simulink model "LF_V15_Delay_Perfect"  (Simulink 7.9)
settings: Solver=ode45  StartTime=0.0  StopTime=100*20e-9  RelTol=1e-3
PreLoadFcn:
  | LF_V15_Param;
values from neighbouring files (symbols this model uses):
  Cnt_CPS = 10    [LF_V15_Param.m]
  Exp_ST = 1/Exp_SF    (= 0.002)    [LF_V15_Param.m]
  Kd2 = 0.004    [LF_V15_Param.m]
  Ki2 = 0.03    [LF_V15_Param.m]
  Kp2 = 0.25    [LF_V15_Param.m]
  Reg_En = (2^Err_Acc_Len)-1    (= 511)    [LF_V15_Param.m]
  Saw_CPS = 100    [LF_V15_Param.m]
libraries: xbsIndex_r4 x273
(part 2 of 2)

== system LF_V15_Delay_Perfect/DC_Direction_Controller/Sampler/Pulse_generator ==
  Freq : Inport
  Accumulator1 : xbsIndex_r4/Accumulator  operation=Add  n_bits=26  overflow=Wrap  scale=1  rst=on  infoeditControl=reset for floating point data type must be asserted for a minimum of 2 cycles  hasbypass=off  en=off  latency=0  dbl_ovrd=off  msb_inp=100  msb=100  lsb=-100  use_behavioral_HDL=on  implementation=Fabric  block_type=accum
  Constant5 : xbsIndex_r4/Constant  const=1/Exp_ST  gui_display_data_type=Fixed-point  arith_type=Unsigned  n_bits=26  bin_pt=0  preci_type=Single  exp_width=8  frac_width=24  explicit_period=on  period=Exp_ST  equ=P=C  opselect=C  inp2=PCIN>>17  opr=+  inp1=P  carry=CIN  dbl_ovrd=off  block_type=constant
  Relational1 : xbsIndex_r4/Relational  mode=a<=b  en=off  latency=0  dbl_ovrd=off  block_type=relational
  Pulse_Level : Outport
  wires:
  Freq/1 -> Accumulator1/1
  Constant5/1 -> Relational1/1
  Accumulator1/1 -> Relational1/2
  Relational1/1 -> Accumulator1/2, Pulse_Level/1

== system LF_V15_Delay_Perfect/DC_Direction_Controller/Sampler/Subsystem1 ==
  In1 : Inport
  Delay : xbsIndex_r4/Delay  rst=off  infoeditControl=Selection of Reset will increase slice count due to use of real FFs and instead of SRLs  en=off  latency=1  dbl_ovrd=off  reg_retiming=on  block_type=delay
  Inverter : xbsIndex_r4/Inverter  en=off  latency=0  dbl_ovrd=off  block_type=inv
  Logical : xbsIndex_r4/Logical  logical_function=AND  inputs=2  en=off  latency=0  precision=User Defined  arith_type=Unsigned  n_bits=1  bin_pt=0  align_bp=on  dbl_ovrd=off  block_type=logical
  Out1 : Outport
  wires:
  Delay/1 -> Logical/2
  Inverter/1 -> Delay/1
  In1/1 -> Logical/1, Inverter/1
  Logical/1 -> Out1/1

== system LF_V15_Delay_Perfect/RM_LM : Actuators/RM_LM: F_R_PWM_Generator/Sawtooth_generator ==
  Freq : Inport
  Accumulator1 : xbsIndex_r4/Accumulator  operation=Add  n_bits=28  overflow=Wrap  scale=1  rst=on  infoeditControl=reset for floating point data type must be asserted for a minimum of 2 cycles  hasbypass=off  en=off  latency=0  dbl_ovrd=off  msb_inp=100  msb=100  lsb=-100  use_behavioral_HDL=on  implementation=Fabric  block_type=accum
  Constant5 : xbsIndex_r4/Constant  const=1/Exp_ST  gui_display_data_type=Fixed-point  arith_type=Unsigned  n_bits=27  bin_pt=0  preci_type=Single  exp_width=8  frac_width=24  explicit_period=on  period=Exp_ST  equ=P=C  opselect=C  inp2=PCIN>>17  opr=+  inp1=P  carry=CIN  dbl_ovrd=off  block_type=constant
  Relational1 : xbsIndex_r4/Relational  mode=a<=b  en=off  latency=0  dbl_ovrd=off  block_type=relational
  Scaling_to_1 : xbsIndex_r4/CMult  const=Exp_ST  gui_display_data_type=Fixed-point  const_n_bits=43  const_bin_pt=43  float_type=Single  exp_bits=8  fraction_bits=24  en=off  latency=0  precision=User Defined  arith_type=Unsigned  n_bits=21  bin_pt=20  quantization=Truncate  overflow=Wrap  dbl_ovrd=off  use_behavioral_HDL=on  mem_type=Distributed RAM  pipeline=off  block_type=cmult
  Sawtooth : Outport
  wires:
  Relational1/1 -> Accumulator1/2
  Accumulator1/1 -> Relational1/2, Scaling_to_1/1
  Constant5/1 -> Relational1/1
  Freq/1 -> Accumulator1/1
  Scaling_to_1/1 -> Sawtooth/1

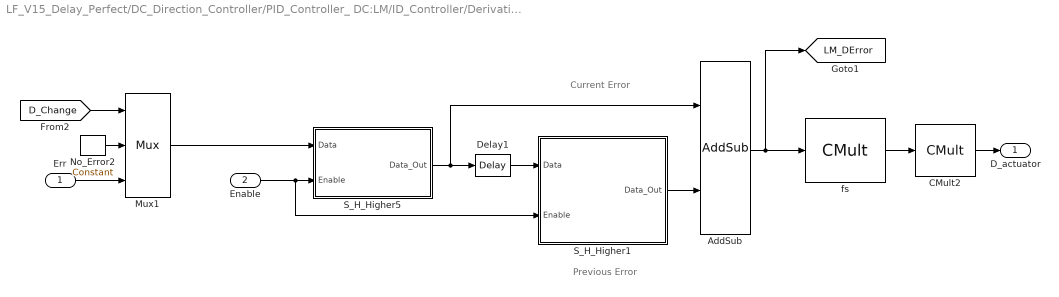
== system LF_V15_Delay_Perfect/DC_Direction_Controller/PID_Controller_ DC:LM/ID_Controller/Derivative ==
  note: Current Error
  note: Previous Error
  Err : Inport
  Enable : Inport  Port=2
  AddSub : xbsIndex_r4/AddSub  mode=Subtraction  use_carryin=off  use_carryout=off  en=off  latency=0  precision=User Defined  arith_type="Signed  (2's comp)"  n_bits=5  bin_pt=0  quantization=Truncate  overflow=Wrap  dbl_ovrd=off  use_behavioral_HDL=off  hw_selection=Fabric  pipelined=off  block_type=addsub
  CMult2 : xbsIndex_r4/CMult  const=Kd2  gui_display_data_type=Fixed-point  const_n_bits=8  const_bin_pt=8  float_type=Single  exp_bits=8  fraction_bits=24  en=off  latency=0  precision=User Defined  arith_type="Signed  (2's comp)"  n_bits=12  bin_pt=12  quantization=Truncate  overflow=Wrap  dbl_ovrd=off  use_behavioral_HDL=off  mem_type=Distributed RAM  pipeline=off  block_type=cmult
  Delay1 : xbsIndex_r4/Delay  rst=off  infoeditControl=Selection of Reset will increase slice count due to use of real FFs and instead of SRLs  en=off  latency=1  dbl_ovrd=off  reg_retiming=off  block_type=delay
  Mux1 : xbsIndex_r4/Mux  inputs=2  en=off  latency=0  precision=Full  arith_type="Signed  (2's comp)"  n_bits=25  bin_pt=20  quantization=Truncate  overflow=Wrap  dbl_ovrd=off  block_type=mux
  No_Error2 : xbsIndex_r4/Constant  const=0  gui_display_data_type=Fixed-point  arith_type=Unsigned  n_bits=1  bin_pt=0  preci_type=Single  exp_width=8  frac_width=24  explicit_period=on  period=Exp_ST  equ=P=C  opselect=C  inp2=PCIN>>17  opr=+  inp1=P  carry=CIN  dbl_ovrd=off  block_type=constant
  S_H_Higher1 : Subsystem
  S_H_Higher5 : Subsystem
  fs : xbsIndex_r4/CMult  const=Cnt_CPS  gui_display_data_type=Fixed-point  const_n_bits=4  const_bin_pt=0  float_type=Single  exp_bits=8  fraction_bits=24  en=off  latency=0  precision=User Defined  arith_type="Signed  (2's comp)"  n_bits=8  bin_pt=0  quantization=Truncate  overflow=Wrap  dbl_ovrd=off  use_behavioral_HDL=on  mem_type=Distributed RAM  pipeline=off  block_type=cmult
  D_actuator : Outport
  tag scope: LM_DError=global
  wires:
  CMult2/1 -> D_actuator/1
  fs/1 -> CMult2/1
  S_H_Higher5/1(Data_Out) -> AddSub/1, Delay1/1
  Enable/1 -> S_H_Higher1/2(Enable), S_H_Higher5/2(Enable)
  Delay1/1 -> S_H_Higher1/1(Data)
  S_H_Higher1/1(Data_Out) -> AddSub/2
  AddSub/1 -> fs/1, [LM_DError]
  [D_Change] -> Mux1/1
  Err/1 -> Mux1/3
  Mux1/1 -> S_H_Higher5/1(Data)
  No_Error2/1 -> Mux1/2

== system LF_V15_Delay_Perfect/DC_Direction_Controller/PID_Controller_ DC:LM/ID_Controller/Integral ==
  Err : Inport
  Enable : Inport  Port=2
  10_Bit_FIFO_Accumulator : Subsystem
  CMult1 : xbsIndex_r4/CMult  const=1/Cnt_CPS  gui_display_data_type=Fixed-point  const_n_bits=40  const_bin_pt=40  float_type=Single  exp_bits=8  fraction_bits=24  en=off  latency=0  precision=User Defined  arith_type="Signed  (2's comp)"  n_bits=17  bin_pt=12  quantization=Truncate  overflow=Wrap  dbl_ovrd=off  use_behavioral_HDL=off  mem_type=Distributed RAM  pipeline=off  block_type=cmult
  Ki2 : xbsIndex_r4/CMult  const=Ki2  gui_display_data_type=Fixed-point  const_n_bits=8  const_bin_pt=8  float_type=Single  exp_bits=8  fraction_bits=24  en=off  latency=0  precision=User Defined  arith_type="Signed  (2's comp)"  n_bits=15  bin_pt=12  quantization=Truncate  overflow=Wrap  dbl_ovrd=off  use_behavioral_HDL=on  mem_type=Distributed RAM  pipeline=off  block_type=cmult
  Mux1 : xbsIndex_r4/Mux  inputs=2  en=off  latency=0  precision=Full  arith_type="Signed  (2's comp)"  n_bits=25  bin_pt=20  quantization=Truncate  overflow=Wrap  dbl_ovrd=off  block_type=mux
  Mux2 : xbsIndex_r4/Mux  inputs=2  en=off  latency=0  precision=Full  arith_type="Signed  (2's comp)"  n_bits=25  bin_pt=20  quantization=Truncate  overflow=Wrap  dbl_ovrd=off  block_type=mux
  No_Error2 : xbsIndex_r4/Constant  const=0  gui_display_data_type=Fixed-point  arith_type=Unsigned  n_bits=1  bin_pt=0  preci_type=Single  exp_width=8  frac_width=24  explicit_period=on  period=Exp_ST  equ=P=C  opselect=C  inp2=PCIN>>17  opr=+  inp1=P  carry=CIN  dbl_ovrd=off  block_type=constant
  ips1 : xbsIndex_r4/Constant  const=0  gui_display_data_type=Fixed-point  arith_type=Unsigned  n_bits=1  bin_pt=0  preci_type=Single  exp_width=8  frac_width=24  explicit_period=on  period=Exp_ST  equ=P=C  opselect=C  inp2=PCIN>>17  opr=+  inp1=P  carry=CIN  dbl_ovrd=off  block_type=constant
  I Actuator : Outport
  tag scope: LM_IError=global
  wires:
  ips1/1 -> Mux2/2
  [In_Ret] -> Mux2/1
  Mux2/1 -> [LM_IError], CMult1/1
  10_Bit_FIFO_Accumulator/1(Error_10_Sum) -> Mux2/3
  [I_Change] -> Mux1/1
  CMult1/1 -> Ki2/1
  Enable/1 -> 10_Bit_FIFO_Accumulator/2(Enable)
  Ki2/1 -> I Actuator/1
  Mux1/1 -> 10_Bit_FIFO_Accumulator/1(Err)
  Err/1 -> Mux1/3
  No_Error2/1 -> Mux1/2

== system LF_V15_Delay_Perfect/DC_Direction_Controller/PID_Controller_ DC:RM/ID_Controller/Derivative ==
  note: Current Error
  note: Previous Error
  Err : Inport
  Enable : Inport  Port=2
  AddSub : xbsIndex_r4/AddSub  mode=Subtraction  use_carryin=off  use_carryout=off  en=off  latency=0  precision=User Defined  arith_type="Signed  (2's comp)"  n_bits=5  bin_pt=0  quantization=Truncate  overflow=Wrap  dbl_ovrd=off  use_behavioral_HDL=off  hw_selection=Fabric  pipelined=off  block_type=addsub
  CMult2 : xbsIndex_r4/CMult  const=Kd2  gui_display_data_type=Fixed-point  const_n_bits=8  const_bin_pt=8  float_type=Single  exp_bits=8  fraction_bits=24  en=off  latency=0  precision=User Defined  arith_type="Signed  (2's comp)"  n_bits=12  bin_pt=12  quantization=Truncate  overflow=Wrap  dbl_ovrd=off  use_behavioral_HDL=off  mem_type=Distributed RAM  pipeline=off  block_type=cmult
  Delay1 : xbsIndex_r4/Delay  rst=off  infoeditControl=Selection of Reset will increase slice count due to use of real FFs and instead of SRLs  en=off  latency=1  dbl_ovrd=off  reg_retiming=off  block_type=delay
  Mux1 : xbsIndex_r4/Mux  inputs=2  en=off  latency=0  precision=Full  arith_type="Signed  (2's comp)"  n_bits=25  bin_pt=20  quantization=Truncate  overflow=Wrap  dbl_ovrd=off  block_type=mux
  No_Error2 : xbsIndex_r4/Constant  const=0  gui_display_data_type=Fixed-point  arith_type=Unsigned  n_bits=1  bin_pt=0  preci_type=Single  exp_width=8  frac_width=24  explicit_period=on  period=Exp_ST  equ=P=C  opselect=C  inp2=PCIN>>17  opr=+  inp1=P  carry=CIN  dbl_ovrd=off  block_type=constant
  S_H_Higher1 : Subsystem
  S_H_Higher5 : Subsystem
  fs : xbsIndex_r4/CMult  const=Cnt_CPS  gui_display_data_type=Fixed-point  const_n_bits=4  const_bin_pt=0  float_type=Single  exp_bits=8  fraction_bits=24  en=off  latency=0  precision=User Defined  arith_type="Signed  (2's comp)"  n_bits=8  bin_pt=0  quantization=Truncate  overflow=Wrap  dbl_ovrd=off  use_behavioral_HDL=on  mem_type=Distributed RAM  pipeline=off  block_type=cmult
  D_actuator : Outport
  tag scope: RM_DError=global
  wires:
  CMult2/1 -> D_actuator/1
  fs/1 -> CMult2/1
  S_H_Higher5/1(Data_Out) -> AddSub/1, Delay1/1
  Enable/1 -> S_H_Higher1/2(Enable), S_H_Higher5/2(Enable)
  Delay1/1 -> S_H_Higher1/1(Data)
  S_H_Higher1/1(Data_Out) -> AddSub/2
  AddSub/1 -> fs/1, [RM_DError]
  [D_Change] -> Mux1/1
  Err/1 -> Mux1/3
  Mux1/1 -> S_H_Higher5/1(Data)
  No_Error2/1 -> Mux1/2

== system LF_V15_Delay_Perfect/DC_Direction_Controller/PID_Controller_ DC:RM/ID_Controller/Integral ==
  Err : Inport
  Enable : Inport  Port=2
  10_Bit_FIFO_Accumulator : Subsystem
  CMult1 : xbsIndex_r4/CMult  const=1/Cnt_CPS  gui_display_data_type=Fixed-point  const_n_bits=40  const_bin_pt=40  float_type=Single  exp_bits=8  fraction_bits=24  en=off  latency=0  precision=User Defined  arith_type="Signed  (2's comp)"  n_bits=17  bin_pt=12  quantization=Truncate  overflow=Wrap  dbl_ovrd=off  use_behavioral_HDL=off  mem_type=Distributed RAM  pipeline=off  block_type=cmult
  Ki2 : xbsIndex_r4/CMult  const=Ki2  gui_display_data_type=Fixed-point  const_n_bits=8  const_bin_pt=8  float_type=Single  exp_bits=8  fraction_bits=24  en=off  latency=0  precision=User Defined  arith_type="Signed  (2's comp)"  n_bits=15  bin_pt=12  quantization=Truncate  overflow=Wrap  dbl_ovrd=off  use_behavioral_HDL=on  mem_type=Distributed RAM  pipeline=off  block_type=cmult
  Mux1 : xbsIndex_r4/Mux  inputs=2  en=off  latency=0  precision=Full  arith_type="Signed  (2's comp)"  n_bits=25  bin_pt=20  quantization=Truncate  overflow=Wrap  dbl_ovrd=off  block_type=mux
  Mux2 : xbsIndex_r4/Mux  inputs=2  en=off  latency=0  precision=Full  arith_type="Signed  (2's comp)"  n_bits=25  bin_pt=20  quantization=Truncate  overflow=Wrap  dbl_ovrd=off  block_type=mux
  No_Error2 : xbsIndex_r4/Constant  const=0  gui_display_data_type=Fixed-point  arith_type=Unsigned  n_bits=1  bin_pt=0  preci_type=Single  exp_width=8  frac_width=24  explicit_period=on  period=Exp_ST  equ=P=C  opselect=C  inp2=PCIN>>17  opr=+  inp1=P  carry=CIN  dbl_ovrd=off  block_type=constant
  ips1 : xbsIndex_r4/Constant  const=0  gui_display_data_type=Fixed-point  arith_type=Unsigned  n_bits=1  bin_pt=0  preci_type=Single  exp_width=8  frac_width=24  explicit_period=on  period=Exp_ST  equ=P=C  opselect=C  inp2=PCIN>>17  opr=+  inp1=P  carry=CIN  dbl_ovrd=off  block_type=constant
  I Actuator : Outport
  tag scope: RM_IError=global
  wires:
  Mux2/1 -> [RM_IError], CMult1/1
  10_Bit_FIFO_Accumulator/1(Error_10_Sum) -> Mux2/3
  [I_Change] -> Mux1/1
  CMult1/1 -> Ki2/1
  Enable/1 -> 10_Bit_FIFO_Accumulator/2(Enable)
  Ki2/1 -> I Actuator/1
  Mux1/1 -> 10_Bit_FIFO_Accumulator/1(Err)
  Err/1 -> Mux1/3
  No_Error2/1 -> Mux1/2
  ips1/1 -> Mux2/2
  [In_Ret] -> Mux2/1

== system LF_V15_Delay_Perfect/DC_Direction_Controller/PID_Controller_ DC:LM/ID_Controller/Derivative/S_H_Higher1 ==
  Data : Inport
  Enable : Inport  Port=2
  Delay2 : xbsIndex_r4/Delay  rst=off  infoeditControl=Selection of Reset will increase slice count due to use of real FFs and instead of SRLs  en=off  latency=1  dbl_ovrd=off  reg_retiming=off  block_type=delay
  Inverter3 : xbsIndex_r4/Inverter  en=off  latency=0  dbl_ovrd=off  block_type=inv
  Mux2 : xbsIndex_r4/Mux  inputs=2  en=off  latency=0  precision=Full  arith_type=Unsigned  n_bits=16  bin_pt=14  quantization=Truncate  overflow=Wrap  dbl_ovrd=off  block_type=mux
  Data_Out : Outport
  wires:
  Data/1 -> Mux2/2
  Mux2/1 -> Delay2/1, Data_Out/1
  Delay2/1 -> Mux2/3
  Inverter3/1 -> Mux2/1
  Enable/1 -> Inverter3/1

== system LF_V15_Delay_Perfect/DC_Direction_Controller/PID_Controller_ DC:LM/ID_Controller/Derivative/S_H_Higher5 ==
  Data : Inport
  Enable : Inport  Port=2
  Delay2 : xbsIndex_r4/Delay  rst=off  infoeditControl=Selection of Reset will increase slice count due to use of real FFs and instead of SRLs  en=off  latency=1  dbl_ovrd=off  reg_retiming=off  block_type=delay
  Inverter3 : xbsIndex_r4/Inverter  en=off  latency=0  dbl_ovrd=off  block_type=inv
  Mux2 : xbsIndex_r4/Mux  inputs=2  en=off  latency=0  precision=Full  arith_type=Unsigned  n_bits=16  bin_pt=14  quantization=Truncate  overflow=Wrap  dbl_ovrd=off  block_type=mux
  Data_Out : Outport
  wires:
  Enable/1 -> Inverter3/1
  Inverter3/1 -> Mux2/1
  Delay2/1 -> Mux2/3
  Mux2/1 -> Data_Out/1, Delay2/1
  Data/1 -> Mux2/2

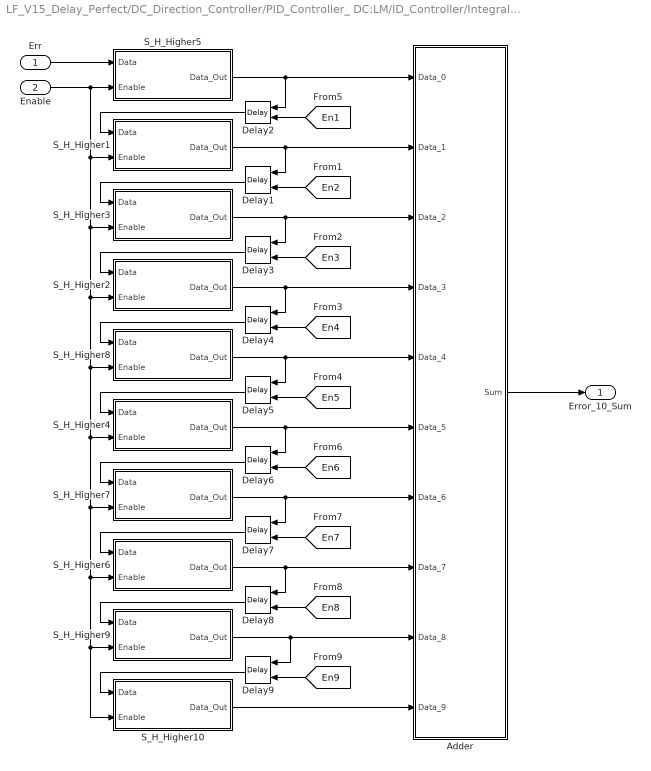
== system LF_V15_Delay_Perfect/DC_Direction_Controller/PID_Controller_ DC:LM/ID_Controller/Integral/10_Bit_FIFO_Accumulator ==
  Err : Inport
  Enable : Inport  Port=2
  Adder : Subsystem
  Delay{1..9} (9 alike) : xbsIndex_r4/Delay  rst=off  infoeditControl=Selection of Reset will increase slice count due to use of real FFs and instead of SRLs  en=on  latency=1  dbl_ovrd=off  reg_retiming=off  block_type=delay
  S_H_Higher1 : Subsystem
  S_H_Higher10 : Subsystem
  S_H_Higher2 : Subsystem
  S_H_Higher3 : Subsystem
  S_H_Higher4 : Subsystem
  S_H_Higher5 : Subsystem
  S_H_Higher6 : Subsystem
  S_H_Higher7 : Subsystem
  S_H_Higher8 : Subsystem
  S_H_Higher9 : Subsystem
  Error_10_Sum : Outport
  wires:
  [En3] -> Delay3/2
  [En4] -> Delay4/2
  [En5] -> Delay5/2
  [En6] -> Delay6/2
  [En7] -> Delay7/2
  [En8] -> Delay8/2
  [En9] -> Delay9/2
  [En2] -> Delay1/2
  [En1] -> Delay2/2
  Delay9/1 -> S_H_Higher10/1(Data)
  S_H_Higher10/1(Data_Out) -> Adder/10(Data_9)
  S_H_Higher9/1(Data_Out) -> Delay9/1, Adder/9(Data_8)
  Delay8/1 -> S_H_Higher9/1(Data)
  S_H_Higher6/1(Data_Out) -> Adder/8(Data_7), Delay8/1
  Err/1 -> S_H_Higher5/1(Data)
  Adder/1(Sum) -> Error_10_Sum/1
  Enable/1 -> S_H_Higher5/2(Enable), S_H_Higher1/2(Enable), S_H_Higher3/2(Enable), S_H_Higher2/2(Enable), S_H_Higher8/2(Enable), S_H_Higher4/2(Enable), S_H_Higher10/2(Enable), S_H_Higher9/2(Enable), S_H_Higher6/2(Enable), S_H_Higher7/2(Enable)
  S_H_Higher3/1(Data_Out) -> Delay3/1, Adder/3(Data_2)
  S_H_Higher2/1(Data_Out) -> Delay4/1, Adder/4(Data_3)
  S_H_Higher8/1(Data_Out) -> Delay5/1, Adder/5(Data_4)
  S_H_Higher4/1(Data_Out) -> Delay6/1, Adder/6(Data_5)
  S_H_Higher7/1(Data_Out) -> Delay7/1, Adder/7(Data_6)
  S_H_Higher5/1(Data_Out) -> Delay2/1, Adder/1(Data_0)
  S_H_Higher1/1(Data_Out) -> Delay1/1, Adder/2(Data_1)
  Delay2/1 -> S_H_Higher1/1(Data)
  Delay1/1 -> S_H_Higher3/1(Data)
  Delay3/1 -> S_H_Higher2/1(Data)
  Delay4/1 -> S_H_Higher8/1(Data)
  Delay5/1 -> S_H_Higher4/1(Data)
  Delay6/1 -> S_H_Higher7/1(Data)
  Delay7/1 -> S_H_Higher6/1(Data)

== system LF_V15_Delay_Perfect/DC_Direction_Controller/PID_Controller_ DC:RM/ID_Controller/Derivative/S_H_Higher1 ==
  Data : Inport
  Enable : Inport  Port=2
  Delay2 : xbsIndex_r4/Delay  rst=off  infoeditControl=Selection of Reset will increase slice count due to use of real FFs and instead of SRLs  en=off  latency=1  dbl_ovrd=off  reg_retiming=off  block_type=delay
  Inverter3 : xbsIndex_r4/Inverter  en=off  latency=0  dbl_ovrd=off  block_type=inv
  Mux2 : xbsIndex_r4/Mux  inputs=2  en=off  latency=0  precision=Full  arith_type=Unsigned  n_bits=16  bin_pt=14  quantization=Truncate  overflow=Wrap  dbl_ovrd=off  block_type=mux
  Data_Out : Outport
  wires:
  Data/1 -> Mux2/2
  Mux2/1 -> Delay2/1, Data_Out/1
  Delay2/1 -> Mux2/3
  Inverter3/1 -> Mux2/1
  Enable/1 -> Inverter3/1

== system LF_V15_Delay_Perfect/DC_Direction_Controller/PID_Controller_ DC:RM/ID_Controller/Derivative/S_H_Higher5 ==
  Data : Inport
  Enable : Inport  Port=2
  Delay2 : xbsIndex_r4/Delay  rst=off  infoeditControl=Selection of Reset will increase slice count due to use of real FFs and instead of SRLs  en=off  latency=1  dbl_ovrd=off  reg_retiming=off  block_type=delay
  Inverter3 : xbsIndex_r4/Inverter  en=off  latency=0  dbl_ovrd=off  block_type=inv
  Mux2 : xbsIndex_r4/Mux  inputs=2  en=off  latency=0  precision=Full  arith_type=Unsigned  n_bits=16  bin_pt=14  quantization=Truncate  overflow=Wrap  dbl_ovrd=off  block_type=mux
  Data_Out : Outport
  wires:
  Enable/1 -> Inverter3/1
  Inverter3/1 -> Mux2/1
  Delay2/1 -> Mux2/3
  Mux2/1 -> Data_Out/1, Delay2/1
  Data/1 -> Mux2/2

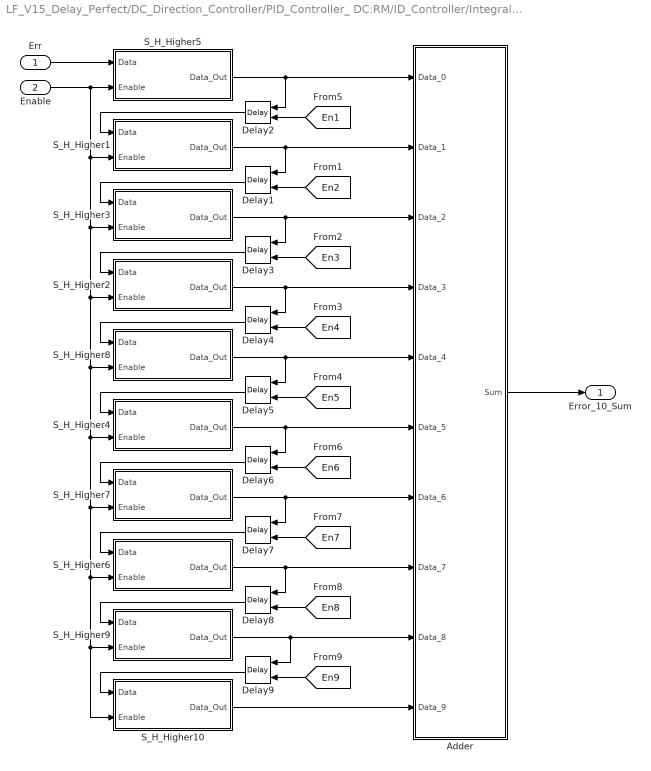
== system LF_V15_Delay_Perfect/DC_Direction_Controller/PID_Controller_ DC:RM/ID_Controller/Integral/10_Bit_FIFO_Accumulator ==
  Err : Inport
  Enable : Inport  Port=2
  Adder : Subsystem
  Delay{1..9} (9 alike) : xbsIndex_r4/Delay  rst=off  infoeditControl=Selection of Reset will increase slice count due to use of real FFs and instead of SRLs  en=on  latency=1  dbl_ovrd=off  reg_retiming=off  block_type=delay
  S_H_Higher1 : Subsystem
  S_H_Higher10 : Subsystem
  S_H_Higher2 : Subsystem
  S_H_Higher3 : Subsystem
  S_H_Higher4 : Subsystem
  S_H_Higher5 : Subsystem
  S_H_Higher6 : Subsystem
  S_H_Higher7 : Subsystem
  S_H_Higher8 : Subsystem
  S_H_Higher9 : Subsystem
  Error_10_Sum : Outport
  wires:
  [En3] -> Delay3/2
  [En4] -> Delay4/2
  [En5] -> Delay5/2
  [En6] -> Delay6/2
  [En7] -> Delay7/2
  [En8] -> Delay8/2
  [En9] -> Delay9/2
  [En2] -> Delay1/2
  [En1] -> Delay2/2
  Delay9/1 -> S_H_Higher10/1(Data)
  S_H_Higher10/1(Data_Out) -> Adder/10(Data_9)
  S_H_Higher9/1(Data_Out) -> Delay9/1, Adder/9(Data_8)
  Delay8/1 -> S_H_Higher9/1(Data)
  S_H_Higher6/1(Data_Out) -> Adder/8(Data_7), Delay8/1
  Err/1 -> S_H_Higher5/1(Data)
  Adder/1(Sum) -> Error_10_Sum/1
  Enable/1 -> S_H_Higher5/2(Enable), S_H_Higher1/2(Enable), S_H_Higher3/2(Enable), S_H_Higher2/2(Enable), S_H_Higher8/2(Enable), S_H_Higher4/2(Enable), S_H_Higher10/2(Enable), S_H_Higher9/2(Enable), S_H_Higher6/2(Enable), S_H_Higher7/2(Enable)
  S_H_Higher3/1(Data_Out) -> Delay3/1, Adder/3(Data_2)
  S_H_Higher2/1(Data_Out) -> Delay4/1, Adder/4(Data_3)
  S_H_Higher8/1(Data_Out) -> Delay5/1, Adder/5(Data_4)
  S_H_Higher4/1(Data_Out) -> Delay6/1, Adder/6(Data_5)
  S_H_Higher7/1(Data_Out) -> Delay7/1, Adder/7(Data_6)
  S_H_Higher5/1(Data_Out) -> Delay2/1, Adder/1(Data_0)
  S_H_Higher1/1(Data_Out) -> Delay1/1, Adder/2(Data_1)
  Delay2/1 -> S_H_Higher1/1(Data)
  Delay1/1 -> S_H_Higher3/1(Data)
  Delay3/1 -> S_H_Higher2/1(Data)
  Delay4/1 -> S_H_Higher8/1(Data)
  Delay5/1 -> S_H_Higher4/1(Data)
  Delay6/1 -> S_H_Higher7/1(Data)
  Delay7/1 -> S_H_Higher6/1(Data)

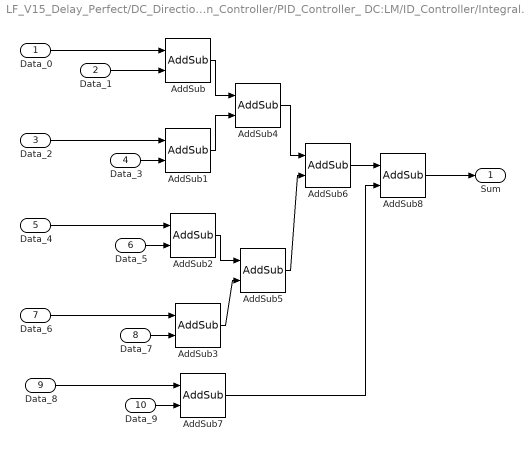
== system LF_V15_Delay_Perfect/DC_Direction_Controller/PID_Controller_ DC:LM/ID_Controller/Integral/10_Bit_FIFO_Accumulator/Adder ==
  Data_0 : Inport
  Data_1 : Inport  Port=2
  Data_2 : Inport  Port=3
  Data_3 : Inport  Port=4
  Data_4 : Inport  Port=5
  Data_5 : Inport  Port=6
  Data_6 : Inport  Port=7
  Data_7 : Inport  Port=8
  Data_8 : Inport  Port=9
  Data_9 : Inport  Port=10
  AddSub{,1..8} (9 alike) : xbsIndex_r4/AddSub  mode=Addition  use_carryin=off  use_carryout=off  en=off  latency=0  precision=Full  arith_type="Signed  (2's comp)"  n_bits=21  bin_pt=11  quantization=Truncate  overflow=Wrap  dbl_ovrd=off  use_behavioral_HDL=off  hw_selection=Fabric  pipelined=off  block_type=addsub
  Sum : Outport
  wires:
  AddSub7/1 -> AddSub8/2
  AddSub6/1 -> AddSub8/1
  AddSub8/1 -> Sum/1
  Data_8/1 -> AddSub7/1
  Data_9/1 -> AddSub7/2
  AddSub/1 -> AddSub4/1
  AddSub1/1 -> AddSub4/2
  AddSub2/1 -> AddSub5/1
  AddSub3/1 -> AddSub5/2
  AddSub4/1 -> AddSub6/1
  AddSub5/1 -> AddSub6/2
  Data_0/1 -> AddSub/1
  Data_1/1 -> AddSub/2
  Data_2/1 -> AddSub1/1
  Data_3/1 -> AddSub1/2
  Data_4/1 -> AddSub2/1
  Data_5/1 -> AddSub2/2
  Data_6/1 -> AddSub3/1
  Data_7/1 -> AddSub3/2

== system LF_V15_Delay_Perfect/DC_Direction_Controller/PID_Controller_ DC:LM/ID_Controller/Integral/10_Bit_FIFO_Accumulator/S_H_Higher1 ==
  Data : Inport
  Enable : Inport  Port=2
  Delay2 : xbsIndex_r4/Delay  rst=off  infoeditControl=Selection of Reset will increase slice count due to use of real FFs and instead of SRLs  en=off  latency=1  dbl_ovrd=off  reg_retiming=off  block_type=delay
  Inverter3 : xbsIndex_r4/Inverter  en=off  latency=0  dbl_ovrd=off  block_type=inv
  Mux2 : xbsIndex_r4/Mux  inputs=2  en=off  latency=0  precision=Full  arith_type=Unsigned  n_bits=16  bin_pt=14  quantization=Truncate  overflow=Wrap  dbl_ovrd=off  block_type=mux
  Data_Out : Outport
  wires:
  Enable/1 -> Inverter3/1
  Inverter3/1 -> Mux2/1
  Delay2/1 -> Mux2/3
  Mux2/1 -> Data_Out/1, Delay2/1
  Data/1 -> Mux2/2

== system LF_V15_Delay_Perfect/DC_Direction_Controller/PID_Controller_ DC:LM/ID_Controller/Integral/10_Bit_FIFO_Accumulator/S_H_Higher10 ==
  Data : Inport
  Enable : Inport  Port=2
  Delay2 : xbsIndex_r4/Delay  rst=off  infoeditControl=Selection of Reset will increase slice count due to use of real FFs and instead of SRLs  en=off  latency=1  dbl_ovrd=off  reg_retiming=off  block_type=delay
  Inverter3 : xbsIndex_r4/Inverter  en=off  latency=0  dbl_ovrd=off  block_type=inv
  Mux2 : xbsIndex_r4/Mux  inputs=2  en=off  latency=0  precision=Full  arith_type=Unsigned  n_bits=16  bin_pt=14  quantization=Truncate  overflow=Wrap  dbl_ovrd=off  block_type=mux
  Data_Out : Outport
  wires:
  Enable/1 -> Inverter3/1
  Inverter3/1 -> Mux2/1
  Delay2/1 -> Mux2/3
  Mux2/1 -> Data_Out/1, Delay2/1
  Data/1 -> Mux2/2

== system LF_V15_Delay_Perfect/DC_Direction_Controller/PID_Controller_ DC:LM/ID_Controller/Integral/10_Bit_FIFO_Accumulator/S_H_Higher2 ==
  Data : Inport
  Enable : Inport  Port=2
  Delay2 : xbsIndex_r4/Delay  rst=off  infoeditControl=Selection of Reset will increase slice count due to use of real FFs and instead of SRLs  en=off  latency=1  dbl_ovrd=off  reg_retiming=off  block_type=delay
  Inverter3 : xbsIndex_r4/Inverter  en=off  latency=0  dbl_ovrd=off  block_type=inv
  Mux2 : xbsIndex_r4/Mux  inputs=2  en=off  latency=0  precision=Full  arith_type=Unsigned  n_bits=16  bin_pt=14  quantization=Truncate  overflow=Wrap  dbl_ovrd=off  block_type=mux
  Data_Out : Outport
  wires:
  Data/1 -> Mux2/2
  Mux2/1 -> Delay2/1, Data_Out/1
  Delay2/1 -> Mux2/3
  Inverter3/1 -> Mux2/1
  Enable/1 -> Inverter3/1

== system LF_V15_Delay_Perfect/DC_Direction_Controller/PID_Controller_ DC:LM/ID_Controller/Integral/10_Bit_FIFO_Accumulator/S_H_Higher3 ==
  Data : Inport
  Enable : Inport  Port=2
  Delay2 : xbsIndex_r4/Delay  rst=off  infoeditControl=Selection of Reset will increase slice count due to use of real FFs and instead of SRLs  en=off  latency=1  dbl_ovrd=off  reg_retiming=off  block_type=delay
  Inverter3 : xbsIndex_r4/Inverter  en=off  latency=0  dbl_ovrd=off  block_type=inv
  Mux2 : xbsIndex_r4/Mux  inputs=2  en=off  latency=0  precision=Full  arith_type=Unsigned  n_bits=16  bin_pt=14  quantization=Truncate  overflow=Wrap  dbl_ovrd=off  block_type=mux
  Data_Out : Outport
  wires:
  Enable/1 -> Inverter3/1
  Inverter3/1 -> Mux2/1
  Delay2/1 -> Mux2/3
  Mux2/1 -> Data_Out/1, Delay2/1
  Data/1 -> Mux2/2

== system LF_V15_Delay_Perfect/DC_Direction_Controller/PID_Controller_ DC:LM/ID_Controller/Integral/10_Bit_FIFO_Accumulator/S_H_Higher4 ==
  Data : Inport
  Enable : Inport  Port=2
  Delay2 : xbsIndex_r4/Delay  rst=off  infoeditControl=Selection of Reset will increase slice count due to use of real FFs and instead of SRLs  en=off  latency=1  dbl_ovrd=off  reg_retiming=off  block_type=delay
  Inverter3 : xbsIndex_r4/Inverter  en=off  latency=0  dbl_ovrd=off  block_type=inv
  Mux2 : xbsIndex_r4/Mux  inputs=2  en=off  latency=0  precision=Full  arith_type=Unsigned  n_bits=16  bin_pt=14  quantization=Truncate  overflow=Wrap  dbl_ovrd=off  block_type=mux
  Data_Out : Outport
  wires:
  Data/1 -> Mux2/2
  Mux2/1 -> Delay2/1, Data_Out/1
  Delay2/1 -> Mux2/3
  Inverter3/1 -> Mux2/1
  Enable/1 -> Inverter3/1

== system LF_V15_Delay_Perfect/DC_Direction_Controller/PID_Controller_ DC:LM/ID_Controller/Integral/10_Bit_FIFO_Accumulator/S_H_Higher5 ==
  Data : Inport
  Enable : Inport  Port=2
  Delay2 : xbsIndex_r4/Delay  rst=off  infoeditControl=Selection of Reset will increase slice count due to use of real FFs and instead of SRLs  en=off  latency=1  dbl_ovrd=off  reg_retiming=off  block_type=delay
  Inverter3 : xbsIndex_r4/Inverter  en=off  latency=0  dbl_ovrd=off  block_type=inv
  Mux2 : xbsIndex_r4/Mux  inputs=2  en=off  latency=0  precision=Full  arith_type=Unsigned  n_bits=16  bin_pt=14  quantization=Truncate  overflow=Wrap  dbl_ovrd=off  block_type=mux
  Data_Out : Outport
  wires:
  Data/1 -> Mux2/2
  Mux2/1 -> Delay2/1, Data_Out/1
  Delay2/1 -> Mux2/3
  Inverter3/1 -> Mux2/1
  Enable/1 -> Inverter3/1

== system LF_V15_Delay_Perfect/DC_Direction_Controller/PID_Controller_ DC:LM/ID_Controller/Integral/10_Bit_FIFO_Accumulator/S_H_Higher6 ==
  Data : Inport
  Enable : Inport  Port=2
  Delay2 : xbsIndex_r4/Delay  rst=off  infoeditControl=Selection of Reset will increase slice count due to use of real FFs and instead of SRLs  en=off  latency=1  dbl_ovrd=off  reg_retiming=off  block_type=delay
  Inverter3 : xbsIndex_r4/Inverter  en=off  latency=0  dbl_ovrd=off  block_type=inv
  Mux2 : xbsIndex_r4/Mux  inputs=2  en=off  latency=0  precision=Full  arith_type=Unsigned  n_bits=16  bin_pt=14  quantization=Truncate  overflow=Wrap  dbl_ovrd=off  block_type=mux
  Data_Out : Outport
  wires:
  Enable/1 -> Inverter3/1
  Inverter3/1 -> Mux2/1
  Delay2/1 -> Mux2/3
  Mux2/1 -> Data_Out/1, Delay2/1
  Data/1 -> Mux2/2

== system LF_V15_Delay_Perfect/DC_Direction_Controller/PID_Controller_ DC:LM/ID_Controller/Integral/10_Bit_FIFO_Accumulator/S_H_Higher7 ==
  Data : Inport
  Enable : Inport  Port=2
  Delay2 : xbsIndex_r4/Delay  rst=off  infoeditControl=Selection of Reset will increase slice count due to use of real FFs and instead of SRLs  en=off  latency=1  dbl_ovrd=off  reg_retiming=off  block_type=delay
  Inverter3 : xbsIndex_r4/Inverter  en=off  latency=0  dbl_ovrd=off  block_type=inv
  Mux2 : xbsIndex_r4/Mux  inputs=2  en=off  latency=0  precision=Full  arith_type=Unsigned  n_bits=16  bin_pt=14  quantization=Truncate  overflow=Wrap  dbl_ovrd=off  block_type=mux
  Data_Out : Outport
  wires:
  Data/1 -> Mux2/2
  Mux2/1 -> Delay2/1, Data_Out/1
  Delay2/1 -> Mux2/3
  Inverter3/1 -> Mux2/1
  Enable/1 -> Inverter3/1

== system LF_V15_Delay_Perfect/DC_Direction_Controller/PID_Controller_ DC:LM/ID_Controller/Integral/10_Bit_FIFO_Accumulator/S_H_Higher8 ==
  Data : Inport
  Enable : Inport  Port=2
  Delay2 : xbsIndex_r4/Delay  rst=off  infoeditControl=Selection of Reset will increase slice count due to use of real FFs and instead of SRLs  en=off  latency=1  dbl_ovrd=off  reg_retiming=off  block_type=delay
  Inverter3 : xbsIndex_r4/Inverter  en=off  latency=0  dbl_ovrd=off  block_type=inv
  Mux2 : xbsIndex_r4/Mux  inputs=2  en=off  latency=0  precision=Full  arith_type=Unsigned  n_bits=16  bin_pt=14  quantization=Truncate  overflow=Wrap  dbl_ovrd=off  block_type=mux
  Data_Out : Outport
  wires:
  Enable/1 -> Inverter3/1
  Inverter3/1 -> Mux2/1
  Delay2/1 -> Mux2/3
  Mux2/1 -> Data_Out/1, Delay2/1
  Data/1 -> Mux2/2

== system LF_V15_Delay_Perfect/DC_Direction_Controller/PID_Controller_ DC:LM/ID_Controller/Integral/10_Bit_FIFO_Accumulator/S_H_Higher9 ==
  Data : Inport
  Enable : Inport  Port=2
  Delay2 : xbsIndex_r4/Delay  rst=off  infoeditControl=Selection of Reset will increase slice count due to use of real FFs and instead of SRLs  en=off  latency=1  dbl_ovrd=off  reg_retiming=off  block_type=delay
  Inverter3 : xbsIndex_r4/Inverter  en=off  latency=0  dbl_ovrd=off  block_type=inv
  Mux2 : xbsIndex_r4/Mux  inputs=2  en=off  latency=0  precision=Full  arith_type=Unsigned  n_bits=16  bin_pt=14  quantization=Truncate  overflow=Wrap  dbl_ovrd=off  block_type=mux
  Data_Out : Outport
  wires:
  Data/1 -> Mux2/2
  Mux2/1 -> Delay2/1, Data_Out/1
  Delay2/1 -> Mux2/3
  Inverter3/1 -> Mux2/1
  Enable/1 -> Inverter3/1

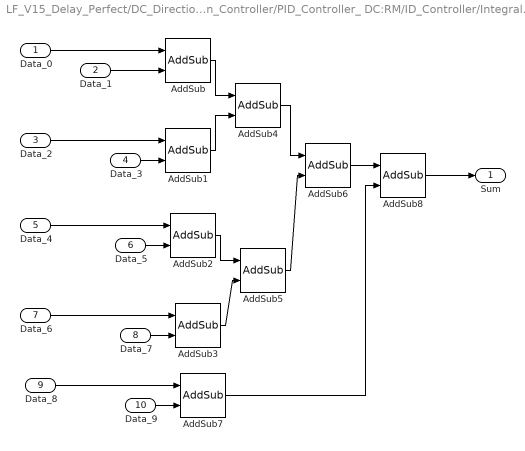
== system LF_V15_Delay_Perfect/DC_Direction_Controller/PID_Controller_ DC:RM/ID_Controller/Integral/10_Bit_FIFO_Accumulator/Adder ==
  Data_0 : Inport
  Data_1 : Inport  Port=2
  Data_2 : Inport  Port=3
  Data_3 : Inport  Port=4
  Data_4 : Inport  Port=5
  Data_5 : Inport  Port=6
  Data_6 : Inport  Port=7
  Data_7 : Inport  Port=8
  Data_8 : Inport  Port=9
  Data_9 : Inport  Port=10
  AddSub{,1..8} (9 alike) : xbsIndex_r4/AddSub  mode=Addition  use_carryin=off  use_carryout=off  en=off  latency=0  precision=Full  arith_type="Signed  (2's comp)"  n_bits=21  bin_pt=11  quantization=Truncate  overflow=Wrap  dbl_ovrd=off  use_behavioral_HDL=off  hw_selection=Fabric  pipelined=off  block_type=addsub
  Sum : Outport
  wires:
  AddSub7/1 -> AddSub8/2
  AddSub6/1 -> AddSub8/1
  AddSub8/1 -> Sum/1
  Data_8/1 -> AddSub7/1
  Data_9/1 -> AddSub7/2
  AddSub/1 -> AddSub4/1
  AddSub1/1 -> AddSub4/2
  AddSub2/1 -> AddSub5/1
  AddSub3/1 -> AddSub5/2
  AddSub4/1 -> AddSub6/1
  AddSub5/1 -> AddSub6/2
  Data_0/1 -> AddSub/1
  Data_1/1 -> AddSub/2
  Data_2/1 -> AddSub1/1
  Data_3/1 -> AddSub1/2
  Data_4/1 -> AddSub2/1
  Data_5/1 -> AddSub2/2
  Data_6/1 -> AddSub3/1
  Data_7/1 -> AddSub3/2

== system LF_V15_Delay_Perfect/DC_Direction_Controller/PID_Controller_ DC:RM/ID_Controller/Integral/10_Bit_FIFO_Accumulator/S_H_Higher1 ==
  Data : Inport
  Enable : Inport  Port=2
  Delay2 : xbsIndex_r4/Delay  rst=off  infoeditControl=Selection of Reset will increase slice count due to use of real FFs and instead of SRLs  en=off  latency=1  dbl_ovrd=off  reg_retiming=off  block_type=delay
  Inverter3 : xbsIndex_r4/Inverter  en=off  latency=0  dbl_ovrd=off  block_type=inv
  Mux2 : xbsIndex_r4/Mux  inputs=2  en=off  latency=0  precision=Full  arith_type=Unsigned  n_bits=16  bin_pt=14  quantization=Truncate  overflow=Wrap  dbl_ovrd=off  block_type=mux
  Data_Out : Outport
  wires:
  Enable/1 -> Inverter3/1
  Inverter3/1 -> Mux2/1
  Delay2/1 -> Mux2/3
  Mux2/1 -> Data_Out/1, Delay2/1
  Data/1 -> Mux2/2

== system LF_V15_Delay_Perfect/DC_Direction_Controller/PID_Controller_ DC:RM/ID_Controller/Integral/10_Bit_FIFO_Accumulator/S_H_Higher10 ==
  Data : Inport
  Enable : Inport  Port=2
  Delay2 : xbsIndex_r4/Delay  rst=off  infoeditControl=Selection of Reset will increase slice count due to use of real FFs and instead of SRLs  en=off  latency=1  dbl_ovrd=off  reg_retiming=off  block_type=delay
  Inverter3 : xbsIndex_r4/Inverter  en=off  latency=0  dbl_ovrd=off  block_type=inv
  Mux2 : xbsIndex_r4/Mux  inputs=2  en=off  latency=0  precision=Full  arith_type=Unsigned  n_bits=16  bin_pt=14  quantization=Truncate  overflow=Wrap  dbl_ovrd=off  block_type=mux
  Data_Out : Outport
  wires:
  Enable/1 -> Inverter3/1
  Inverter3/1 -> Mux2/1
  Delay2/1 -> Mux2/3
  Mux2/1 -> Data_Out/1, Delay2/1
  Data/1 -> Mux2/2

== system LF_V15_Delay_Perfect/DC_Direction_Controller/PID_Controller_ DC:RM/ID_Controller/Integral/10_Bit_FIFO_Accumulator/S_H_Higher2 ==
  Data : Inport
  Enable : Inport  Port=2
  Delay2 : xbsIndex_r4/Delay  rst=off  infoeditControl=Selection of Reset will increase slice count due to use of real FFs and instead of SRLs  en=off  latency=1  dbl_ovrd=off  reg_retiming=off  block_type=delay
  Inverter3 : xbsIndex_r4/Inverter  en=off  latency=0  dbl_ovrd=off  block_type=inv
  Mux2 : xbsIndex_r4/Mux  inputs=2  en=off  latency=0  precision=Full  arith_type=Unsigned  n_bits=16  bin_pt=14  quantization=Truncate  overflow=Wrap  dbl_ovrd=off  block_type=mux
  Data_Out : Outport
  wires:
  Data/1 -> Mux2/2
  Mux2/1 -> Delay2/1, Data_Out/1
  Delay2/1 -> Mux2/3
  Inverter3/1 -> Mux2/1
  Enable/1 -> Inverter3/1

== system LF_V15_Delay_Perfect/DC_Direction_Controller/PID_Controller_ DC:RM/ID_Controller/Integral/10_Bit_FIFO_Accumulator/S_H_Higher3 ==
  Data : Inport
  Enable : Inport  Port=2
  Delay2 : xbsIndex_r4/Delay  rst=off  infoeditControl=Selection of Reset will increase slice count due to use of real FFs and instead of SRLs  en=off  latency=1  dbl_ovrd=off  reg_retiming=off  block_type=delay
  Inverter3 : xbsIndex_r4/Inverter  en=off  latency=0  dbl_ovrd=off  block_type=inv
  Mux2 : xbsIndex_r4/Mux  inputs=2  en=off  latency=0  precision=Full  arith_type=Unsigned  n_bits=16  bin_pt=14  quantization=Truncate  overflow=Wrap  dbl_ovrd=off  block_type=mux
  Data_Out : Outport
  wires:
  Enable/1 -> Inverter3/1
  Inverter3/1 -> Mux2/1
  Delay2/1 -> Mux2/3
  Mux2/1 -> Data_Out/1, Delay2/1
  Data/1 -> Mux2/2

== system LF_V15_Delay_Perfect/DC_Direction_Controller/PID_Controller_ DC:RM/ID_Controller/Integral/10_Bit_FIFO_Accumulator/S_H_Higher4 ==
  Data : Inport
  Enable : Inport  Port=2
  Delay2 : xbsIndex_r4/Delay  rst=off  infoeditControl=Selection of Reset will increase slice count due to use of real FFs and instead of SRLs  en=off  latency=1  dbl_ovrd=off  reg_retiming=off  block_type=delay
  Inverter3 : xbsIndex_r4/Inverter  en=off  latency=0  dbl_ovrd=off  block_type=inv
  Mux2 : xbsIndex_r4/Mux  inputs=2  en=off  latency=0  precision=Full  arith_type=Unsigned  n_bits=16  bin_pt=14  quantization=Truncate  overflow=Wrap  dbl_ovrd=off  block_type=mux
  Data_Out : Outport
  wires:
  Data/1 -> Mux2/2
  Mux2/1 -> Delay2/1, Data_Out/1
  Delay2/1 -> Mux2/3
  Inverter3/1 -> Mux2/1
  Enable/1 -> Inverter3/1

== system LF_V15_Delay_Perfect/DC_Direction_Controller/PID_Controller_ DC:RM/ID_Controller/Integral/10_Bit_FIFO_Accumulator/S_H_Higher5 ==
  Data : Inport
  Enable : Inport  Port=2
  Delay2 : xbsIndex_r4/Delay  rst=off  infoeditControl=Selection of Reset will increase slice count due to use of real FFs and instead of SRLs  en=off  latency=1  dbl_ovrd=off  reg_retiming=off  block_type=delay
  Inverter3 : xbsIndex_r4/Inverter  en=off  latency=0  dbl_ovrd=off  block_type=inv
  Mux2 : xbsIndex_r4/Mux  inputs=2  en=off  latency=0  precision=Full  arith_type=Unsigned  n_bits=16  bin_pt=14  quantization=Truncate  overflow=Wrap  dbl_ovrd=off  block_type=mux
  Data_Out : Outport
  wires:
  Data/1 -> Mux2/2
  Mux2/1 -> Delay2/1, Data_Out/1
  Delay2/1 -> Mux2/3
  Inverter3/1 -> Mux2/1
  Enable/1 -> Inverter3/1

== system LF_V15_Delay_Perfect/DC_Direction_Controller/PID_Controller_ DC:RM/ID_Controller/Integral/10_Bit_FIFO_Accumulator/S_H_Higher6 ==
  Data : Inport
  Enable : Inport  Port=2
  Delay2 : xbsIndex_r4/Delay  rst=off  infoeditControl=Selection of Reset will increase slice count due to use of real FFs and instead of SRLs  en=off  latency=1  dbl_ovrd=off  reg_retiming=off  block_type=delay
  Inverter3 : xbsIndex_r4/Inverter  en=off  latency=0  dbl_ovrd=off  block_type=inv
  Mux2 : xbsIndex_r4/Mux  inputs=2  en=off  latency=0  precision=Full  arith_type=Unsigned  n_bits=16  bin_pt=14  quantization=Truncate  overflow=Wrap  dbl_ovrd=off  block_type=mux
  Data_Out : Outport
  wires:
  Enable/1 -> Inverter3/1
  Inverter3/1 -> Mux2/1
  Delay2/1 -> Mux2/3
  Mux2/1 -> Data_Out/1, Delay2/1
  Data/1 -> Mux2/2

== system LF_V15_Delay_Perfect/DC_Direction_Controller/PID_Controller_ DC:RM/ID_Controller/Integral/10_Bit_FIFO_Accumulator/S_H_Higher7 ==
  Data : Inport
  Enable : Inport  Port=2
  Delay2 : xbsIndex_r4/Delay  rst=off  infoeditControl=Selection of Reset will increase slice count due to use of real FFs and instead of SRLs  en=off  latency=1  dbl_ovrd=off  reg_retiming=off  block_type=delay
  Inverter3 : xbsIndex_r4/Inverter  en=off  latency=0  dbl_ovrd=off  block_type=inv
  Mux2 : xbsIndex_r4/Mux  inputs=2  en=off  latency=0  precision=Full  arith_type=Unsigned  n_bits=16  bin_pt=14  quantization=Truncate  overflow=Wrap  dbl_ovrd=off  block_type=mux
  Data_Out : Outport
  wires:
  Data/1 -> Mux2/2
  Mux2/1 -> Delay2/1, Data_Out/1
  Delay2/1 -> Mux2/3
  Inverter3/1 -> Mux2/1
  Enable/1 -> Inverter3/1

== system LF_V15_Delay_Perfect/DC_Direction_Controller/PID_Controller_ DC:RM/ID_Controller/Integral/10_Bit_FIFO_Accumulator/S_H_Higher8 ==
  Data : Inport
  Enable : Inport  Port=2
  Delay2 : xbsIndex_r4/Delay  rst=off  infoeditControl=Selection of Reset will increase slice count due to use of real FFs and instead of SRLs  en=off  latency=1  dbl_ovrd=off  reg_retiming=off  block_type=delay
  Inverter3 : xbsIndex_r4/Inverter  en=off  latency=0  dbl_ovrd=off  block_type=inv
  Mux2 : xbsIndex_r4/Mux  inputs=2  en=off  latency=0  precision=Full  arith_type=Unsigned  n_bits=16  bin_pt=14  quantization=Truncate  overflow=Wrap  dbl_ovrd=off  block_type=mux
  Data_Out : Outport
  wires:
  Enable/1 -> Inverter3/1
  Inverter3/1 -> Mux2/1
  Delay2/1 -> Mux2/3
  Mux2/1 -> Data_Out/1, Delay2/1
  Data/1 -> Mux2/2

== system LF_V15_Delay_Perfect/DC_Direction_Controller/PID_Controller_ DC:RM/ID_Controller/Integral/10_Bit_FIFO_Accumulator/S_H_Higher9 ==
  Data : Inport
  Enable : Inport  Port=2
  Delay2 : xbsIndex_r4/Delay  rst=off  infoeditControl=Selection of Reset will increase slice count due to use of real FFs and instead of SRLs  en=off  latency=1  dbl_ovrd=off  reg_retiming=off  block_type=delay
  Inverter3 : xbsIndex_r4/Inverter  en=off  latency=0  dbl_ovrd=off  block_type=inv
  Mux2 : xbsIndex_r4/Mux  inputs=2  en=off  latency=0  precision=Full  arith_type=Unsigned  n_bits=16  bin_pt=14  quantization=Truncate  overflow=Wrap  dbl_ovrd=off  block_type=mux
  Data_Out : Outport
  wires:
  Data/1 -> Mux2/2
  Mux2/1 -> Delay2/1, Data_Out/1
  Delay2/1 -> Mux2/3
  Inverter3/1 -> Mux2/1
  Enable/1 -> Inverter3/1
